simulink model "linear_control_sys"  (R2024a)
settings: Solver=VariableStepAuto  StartTime=0.0  StopTime=100  RelTol=1e-3
undefined symbols (not defined in the file or in its folder): den, linsys1, num
settings Model: Creator=gladstonjoseph  LastModifiedBy=gladstonjoseph

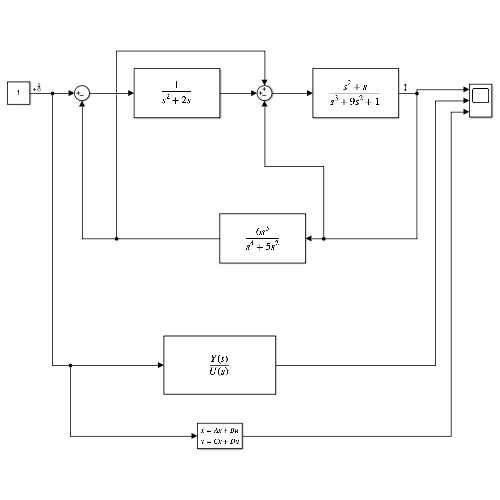
[thumbnail: Simulink's stored preview of the top-level diagram]
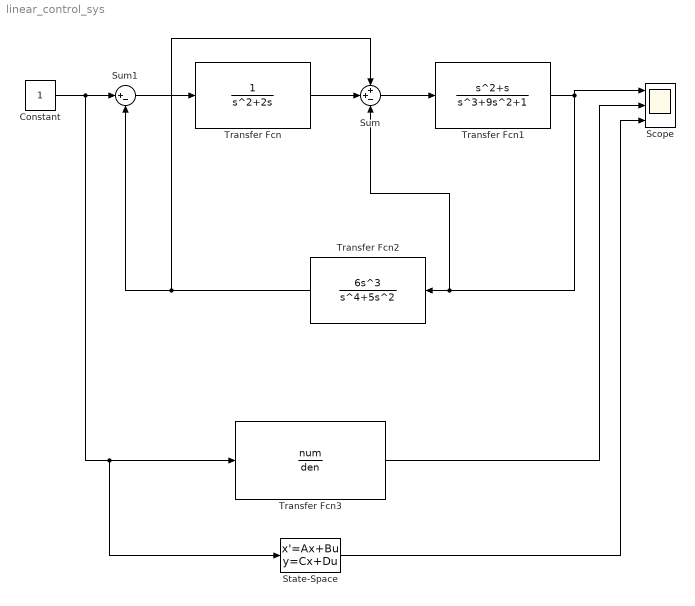
== system linear_control_sys ==
  Constant : Constant
  Scope : Scope  NumInputPorts=3
  State-Space : StateSpace  A=linsys1.A  B=linsys1.B  C=linsys1.C  D=linsys1.D  InitialCondition=0
  Sum : Sum  Inputs=++-
  Sum1 : Sum  Inputs=|+-
  Transfer Fcn : TransferFcn  Denominator=[1 2 0]
  Transfer Fcn1 : TransferFcn  Numerator=[1 1 0]  Denominator=[1 9 0 1]
  Transfer Fcn2 : TransferFcn  Numerator=[6 0 0 0]  Denominator=[1 0 5 0 0]
  Transfer Fcn3 : TransferFcn  Numerator=num  Denominator=den
  wires:
  Transfer Fcn2/1 -> Sum1/2, Sum/1
  Transfer Fcn1/1 -> Scope/1, Sum/3, Transfer Fcn2/1
  Sum/1 -> Transfer Fcn1/1
  Transfer Fcn/1 -> Sum/2
  Sum1/1 -> Transfer Fcn/1
  Constant/1 -> State-Space/1, Transfer Fcn3/1, Sum1/1
  Transfer Fcn3/1 -> Scope/2
  State-Space/1 -> Scope/3
